simulink model "model"  (R2023a)
settings: Solver=VariableStepAuto  StartTime=0.0  StopTime=10  RelTol=1e-3
settings Model: Creator=grill  LastModifiedBy=grill

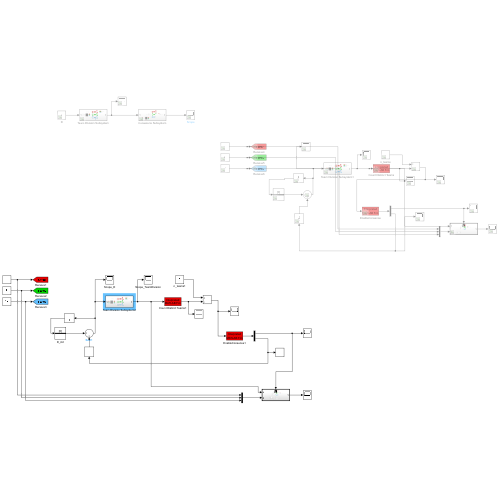
[thumbnail: Simulink's stored preview of the top-level diagram]
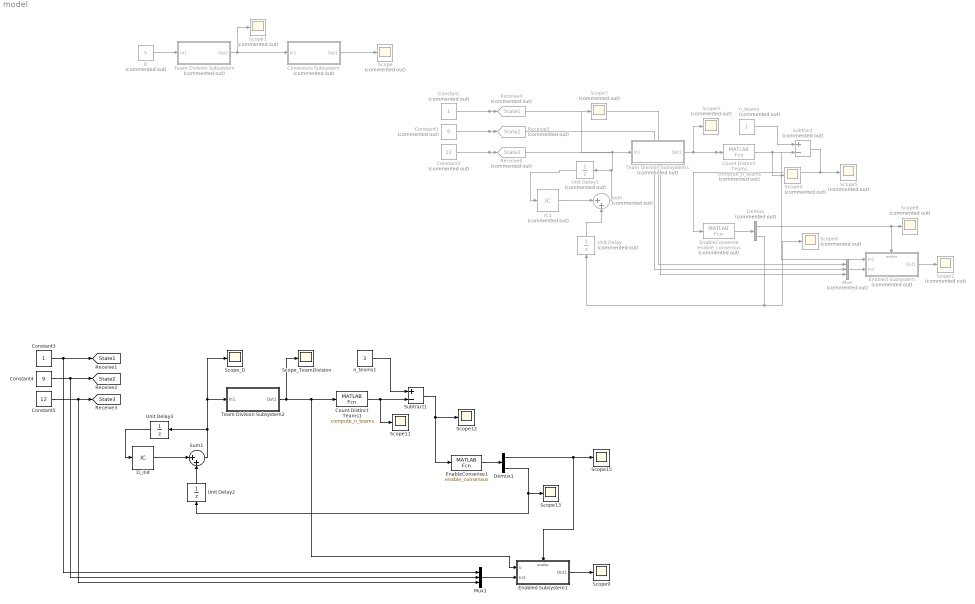
== system model ==
  " Receive4" : Goto  Commented=on  GotoTag=State1  TagVisibility=global
  " Receive5" : Goto  Commented=on  GotoTag=State2  TagVisibility=global
  " Receive6" : Goto  Commented=on  GotoTag=State3  TagVisibility=global
  Consesuns Subsystem : Subsystem  Commented=on
  Constant : Constant  Commented=on
  Constant1 : Constant  Commented=on  Value=9
  Constant2 : Constant  Commented=on  Value=12
  Constant3 : Constant
  Constant4 : Constant  Value=9
  Constant5 : Constant  Value=12
  Count Distinct Teams : MATLABFcn  Commented=on  MATLABFcn=compute_n_teams  OutputDimensions=1
  Count Distinct Teams1 : MATLABFcn  MATLABFcn=compute_n_teams  OutputDimensions=1
  D : Constant  Commented=on  Value=5
  D_init : InitialCondition  Value=0
  Demux : Demux  Commented=on  Outputs=2
  Demux1 : Demux  Outputs=2
  EnableConsense : MATLABFcn  Commented=on  MATLABFcn=enable_consensus  OutputDimensions=2
  EnableConsense1 : MATLABFcn  MATLABFcn=enable_consensus  OutputDimensions=2
  Enabled Subsystem : Subsystem  Commented=on  TreatAsAtomicUnit=on
  Enabled Subsystem1 : Subsystem  TreatAsAtomicUnit=on
  IC1 : InitialCondition  Commented=on  Value=0
  Mux : Mux  Commented=on  Inputs=3
  Mux1 : Mux  Inputs=3
  Scope{,1..8} (9 alike) : Scope  Commented=on
  Scope{9,11..13,15} (5 alike) : Scope
  Scope_D : Scope
  Scope_TeamDivision : Scope
  Subtract : Sum  Commented=on  Inputs=+-
  Subtract1 : Sum  Inputs=+-
  Sum : Sum  Commented=on  Inputs=|++
  Sum1 : Sum  Inputs=|++
  Team Division Subsystem : Subsystem  Commented=on
  Team Division Subsystem1 : Subsystem  Commented=on
  Team Division Subsystem2 : Subsystem
  Unit Delay : UnitDelay  Commented=on  SampleTime=-1  HasFrameUpgradeWarning=on
  Unit Delay1 : UnitDelay  Commented=on  SampleTime=-1  HasFrameUpgradeWarning=on
  Unit Delay2 : UnitDelay  SampleTime=-1  HasFrameUpgradeWarning=on
  Unit Delay3 : UnitDelay  SampleTime=-1  HasFrameUpgradeWarning=on
  n_teams : Constant  Commented=on
  n_teams1 : Constant  Value=3
  tag scope: State1=global, State2=global, State3=global
  wires:
  D/1 -> Team Division Subsystem/1(In1)
  Consesuns Subsystem/1(Out1) -> Scope/1
  Constant/1 -> Mux/1, " Receive4"/1
  Constant1/1 -> Mux/2, " Receive5"/1
  Constant2/1 -> Mux/3, " Receive6"/1
  Team Division Subsystem/1(Out1) -> Scope1/1, Consesuns Subsystem/1(In1)
  Mux/1 -> Enabled Subsystem/2(In2)
  n_teams/1 -> Subtract/1
  Subtract/1 -> Scope5/1, EnableConsense/1
  Count Distinct Teams/1 -> Scope4/1, Subtract/2
  Demux/2 -> Scope6/1, Unit Delay/1
  Team Division Subsystem1/1(Out1) -> Enabled Subsystem/1(In1), Count Distinct Teams/1, Scope3/1
  Unit Delay/1 -> Sum/2
  Sum/1 -> Team Division Subsystem1/1(In1), Scope7/1, Unit Delay1/1
  IC1/1 -> Sum/1
  Unit Delay1/1 -> IC1/1
  EnableConsense/1 -> Demux/1
  Demux/1 -> Scope8/1, Enabled Subsystem/Enable
  Enabled Subsystem/1(Out1) -> Scope2/1
  Demux1/1 -> Scope15/1, Enabled Subsystem1/Enable
  Enabled Subsystem1/1(Out1) -> Scope9/1
  D_init/1 -> Sum1/1
  Unit Delay3/1 -> D_init/1
  EnableConsense1/1 -> Demux1/1
  Team Division Subsystem2/1(Out1) -> Enabled Subsystem1/1(u), Count Distinct Teams1/1, Scope_TeamDivision/1
  Unit Delay2/1 -> Sum1/2
  Constant5/1 -> [State3], Mux1/3
  Constant4/1 -> Mux1/2, [State2]
  Sum1/1 -> Team Division Subsystem2/1(In1), Scope_D/1, Unit Delay3/1
  Subtract1/1 -> EnableConsense1/1, Scope12/1
  Constant3/1 -> [State1], Mux1/1
  n_teams1/1 -> Subtract1/1
  Mux1/1 -> Enabled Subsystem1/2(In2)
  Count Distinct Teams1/1 -> Scope11/1, Subtract1/2
  Demux1/2 -> Unit Delay2/1, Scope13/1

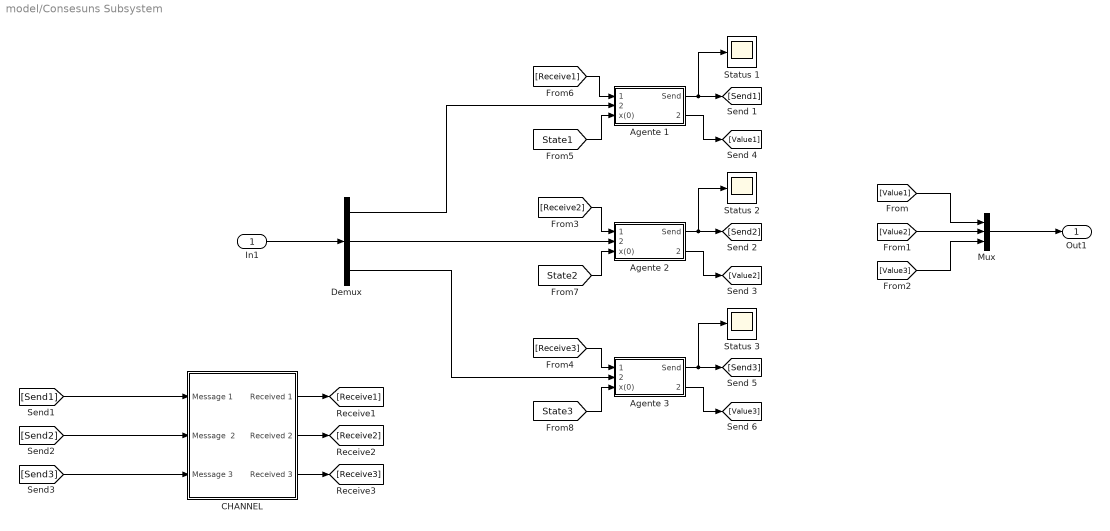
== system model/Consesuns Subsystem ==
  In1 : Inport
  Agente 1 : Subsystem
  Agente 2 : Subsystem
  Agente 3 : Subsystem
  CHANNEL : Subsystem
  Demux : Demux  Outputs=3
  Mux : Mux  Inputs=3
  Status 1 : Scope
  Status 2 : Scope
  Status 3 : Scope
  Out1 : Outport
  wires:
  Agente 1/1(Send) -> [Send1], Status 1/1
  In1/1 -> Demux/1
  Mux/1 -> Out1/1
  [Value3] -> Mux/3
  [Value2] -> Mux/2
  [Value1] -> Mux/1
  Demux/1 -> Agente 1/2(team_id)
  Agente 1/2(ValuePort) -> [Value1]
  Agente 2/1(Send) -> [Send2], Status 2/1
  Demux/2 -> Agente 2/2(team_id)
  Agente 2/2(ValuePort) -> [Value2]
  Agente 3/1(Send) -> [Send3], Status 3/1
  Demux/3 -> Agente 3/2(team_id)
  Agente 3/2(ValuePort) -> [Value3]
  [Receive1] -> Agente 1/1(Receive)
  [Receive2] -> Agente 2/1(Receive)
  [Receive3] -> Agente 3/1(Receive)
  CHANNEL/2(Received 2) -> [Receive2]
  CHANNEL/1(Received 1) -> [Receive1]
  CHANNEL/3(Received 3) -> [Receive3]
  [State1] -> Agente 1/3(x(0))
  [State2] -> Agente 2/3(x(0))
  [State3] -> Agente 3/3(x(0))
  [Send3] -> CHANNEL/3(Message 3)
  [Send2] -> CHANNEL/2(Message  2)
  [Send1] -> CHANNEL/1(Message 1)

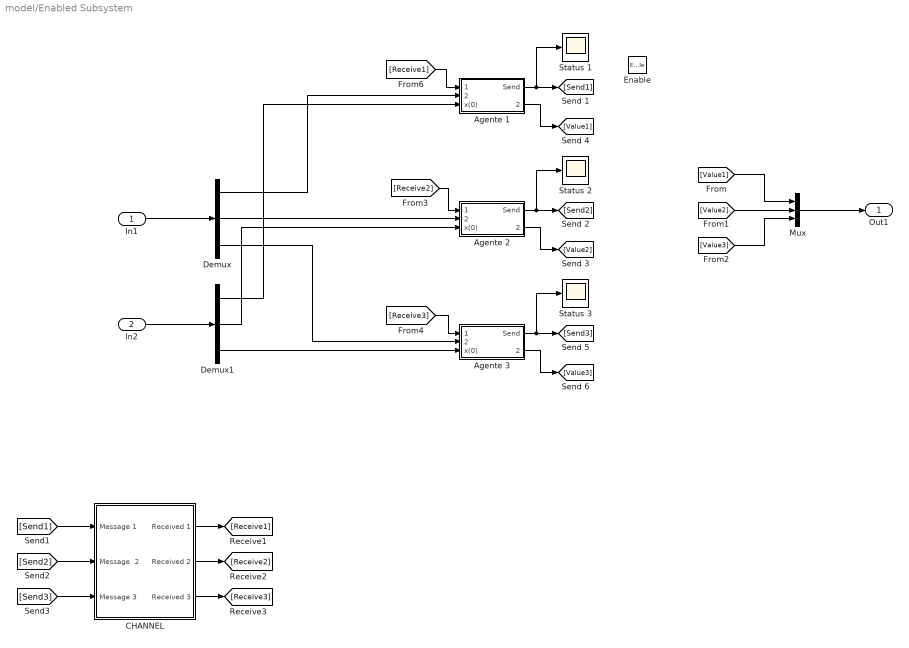
== system model/Enabled Subsystem ==
  In1 : Inport
  In2 : Inport  Port=2
  Enable : EnablePort
  Agente 1 : Subsystem
  Agente 2 : Subsystem
  Agente 3 : Subsystem
  CHANNEL : Subsystem
  Demux : Demux  Outputs=3
  Demux1 : Demux  Outputs=3
  Mux : Mux  Inputs=3
  Status 1 : Scope
  Status 2 : Scope
  Status 3 : Scope
  Out1 : Outport
  wires:
  Demux1/3 -> Agente 3/3(x(0))
  Demux1/1 -> Agente 1/3(x(0))
  Demux/2 -> Agente 2/2(team_id)
  Demux1/2 -> Agente 2/3(x(0))
  Agente 2/1(Send) -> [Send2], Status 2/1
  CHANNEL/3(Received 3) -> [Receive3]
  In1/1 -> Demux/1
  Agente 3/2(ValuePort) -> [Value3]
  [Value3] -> Mux/3
  Agente 2/2(ValuePort) -> [Value2]
  Agente 1/2(ValuePort) -> [Value1]
  [Receive2] -> Agente 2/1(Receive)
  [Receive3] -> Agente 3/1(Receive)
  CHANNEL/2(Received 2) -> [Receive2]
  In2/1 -> Demux1/1
  [Value1] -> Mux/1
  Mux/1 -> Out1/1
  [Send1] -> CHANNEL/1(Message 1)
  [Send2] -> CHANNEL/2(Message  2)
  [Send3] -> CHANNEL/3(Message 3)
  [Receive1] -> Agente 1/1(Receive)
  Demux/1 -> Agente 1/2(team_id)
  [Value2] -> Mux/2
  Agente 1/1(Send) -> [Send1], Status 1/1
  CHANNEL/1(Received 1) -> [Receive1]
  Demux/3 -> Agente 3/2(team_id)
  Agente 3/1(Send) -> [Send3], Status 3/1

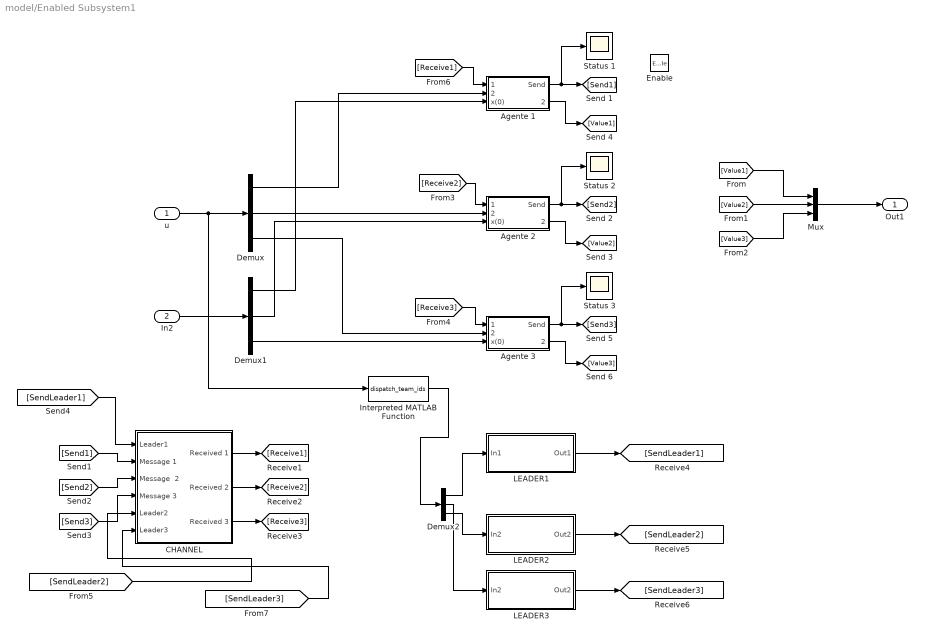
== system model/Enabled Subsystem1 ==
  u : Inport
  In2 : Inport  Port=2
  Enable : EnablePort
  Agente 1 : Subsystem
  Agente 2 : Subsystem
  Agente 3 : Subsystem
  CHANNEL : Subsystem
  Demux : Demux  Outputs=3
  Demux1 : Demux  Outputs=3
  Demux2 : Demux  Outputs=3
  Interpreted MATLAB Function : MATLABFcn  MATLABFcn=dispatch_team_ids  OutputDimensions=3
  LEADER1 : Subsystem
  LEADER2 : Subsystem
  LEADER3 : Subsystem
  Mux : Mux  Inputs=3
  Status 1 : Scope
  Status 2 : Scope
  Status 3 : Scope
  Out1 : Outport
  wires:
  Demux1/3 -> Agente 3/3(x(0))
  Demux1/1 -> Agente 1/3(x(0))
  Demux/2 -> Agente 2/2(team_id)
  Demux1/2 -> Agente 2/3(x(0))
  Agente 2/1(Send) -> [Send2], Status 2/1
  CHANNEL/3(Received 3) -> [Receive3]
  u/1 -> Interpreted MATLAB Function/1, Demux/1
  Agente 3/2(ValuePort) -> [Value3]
  [Value3] -> Mux/3
  Agente 2/2(ValuePort) -> [Value2]
  Agente 1/2(ValuePort) -> [Value1]
  [Receive2] -> Agente 2/1(Receive)
  [Receive3] -> Agente 3/1(Receive)
  CHANNEL/2(Received 2) -> [Receive2]
  In2/1 -> Demux1/1
  [Value1] -> Mux/1
  Mux/1 -> Out1/1
  [Send1] -> CHANNEL/2(Message 1)
  [Send2] -> CHANNEL/3(Message  2)
  [Send3] -> CHANNEL/4(Message 3)
  [Receive1] -> Agente 1/1(Receive)
  Demux/1 -> Agente 1/2(team_id)
  [Value2] -> Mux/2
  Agente 1/1(Send) -> [Send1], Status 1/1
  CHANNEL/1(Received 1) -> [Receive1]
  Demux/3 -> Agente 3/2(team_id)
  Agente 3/1(Send) -> [Send3], Status 3/1
  LEADER1/1(Out1) -> [SendLeader1]
  [SendLeader1] -> CHANNEL/1(Leader1)
  LEADER2/1(Out2) -> [SendLeader2]
  [SendLeader2] -> CHANNEL/5(Leader2)
  Interpreted MATLAB Function/1 -> Demux2/1
  Demux2/1 -> LEADER1/1(In1)
  Demux2/3 -> LEADER2/1(In2)
  LEADER3/1(Out2) -> [SendLeader3]
  Demux2/2 -> LEADER3/1(In2)
  [SendLeader3] -> CHANNEL/6(Leader3)

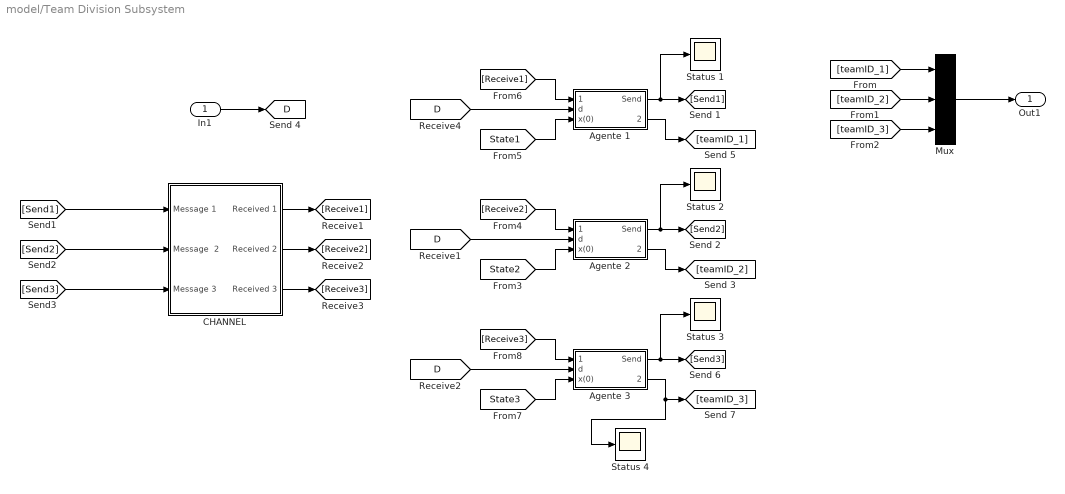
== system model/Team Division Subsystem ==
  In1 : Inport
  Agente 1 : Subsystem
  Agente 2 : Subsystem
  Agente 3 : Subsystem
  CHANNEL : Subsystem
  Mux : Mux  Inputs=3
  Status {1..4} (4 alike) : Scope
  Out1 : Outport
  tag scope: D=global
  wires:
  Agente 1/1(Send) -> [Send1], Status 1/1
  [D] -> Agente 1/2(d)
  Mux/1 -> Out1/1
  Agente 1/2(TeamPort) -> [teamID_1]
  [teamID_3] -> Mux/3
  [teamID_2] -> Mux/2
  [teamID_1] -> Mux/1
  In1/1 -> [D]
  [Receive1] -> Agente 1/1(Receive)
  [State1] -> Agente 1/3(x(0))
  Agente 2/2(TeamPort) -> [teamID_2]
  [State2] -> Agente 2/3(x(0))
  Agente 2/1(Send) -> [Send2], Status 2/1
  [D] -> Agente 2/2(d)
  [Receive2] -> Agente 2/1(Receive)
  Agente 3/2(TeamPort) -> Status 4/1, [teamID_3]
  [State3] -> Agente 3/3(x(0))
  Agente 3/1(Send) -> [Send3], Status 3/1
  [D] -> Agente 3/2(d)
  [Receive3] -> Agente 3/1(Receive)
  CHANNEL/2(Received 2) -> [Receive2]
  CHANNEL/1(Received 1) -> [Receive1]
  CHANNEL/3(Received 3) -> [Receive3]
  [Send1] -> CHANNEL/1(Message 1)
  [Send2] -> CHANNEL/2(Message  2)
  [Send3] -> CHANNEL/3(Message 3)

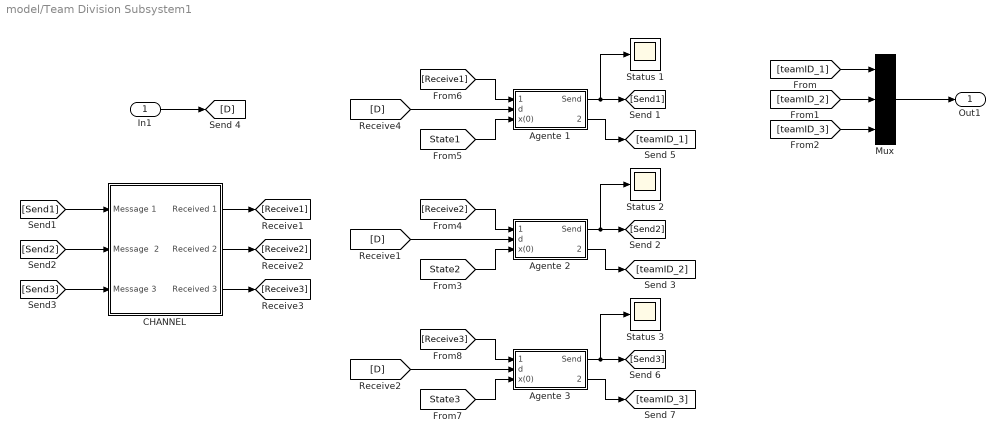
== system model/Team Division Subsystem1 ==
  In1 : Inport
  Agente 1 : Subsystem
  Agente 2 : Subsystem
  Agente 3 : Subsystem
  CHANNEL : Subsystem
  Mux : Mux  Inputs=3
  Status 1 : Scope
  Status 2 : Scope
  Status 3 : Scope
  Out1 : Outport
  wires:
  Agente 1/1(Send) -> [Send1], Status 1/1
  [D] -> Agente 1/2(d)
  Mux/1 -> Out1/1
  Agente 1/2(TeamPort) -> [teamID_1]
  [teamID_3] -> Mux/3
  [teamID_2] -> Mux/2
  [teamID_1] -> Mux/1
  In1/1 -> [D]
  [Receive1] -> Agente 1/1(Receive)
  [State1] -> Agente 1/3(x(0))
  Agente 2/2(TeamPort) -> [teamID_2]
  [State2] -> Agente 2/3(x(0))
  Agente 2/1(Send) -> [Send2], Status 2/1
  [D] -> Agente 2/2(d)
  [Receive2] -> Agente 2/1(Receive)
  Agente 3/2(TeamPort) -> [teamID_3]
  [State3] -> Agente 3/3(x(0))
  Agente 3/1(Send) -> [Send3], Status 3/1
  [D] -> Agente 3/2(d)
  [Receive3] -> Agente 3/1(Receive)
  CHANNEL/2(Received 2) -> [Receive2]
  [Send1] -> CHANNEL/1(Message 1)
  CHANNEL/1(Received 1) -> [Receive1]
  [Send2] -> CHANNEL/2(Message  2)
  [Send3] -> CHANNEL/3(Message 3)
  CHANNEL/3(Received 3) -> [Receive3]

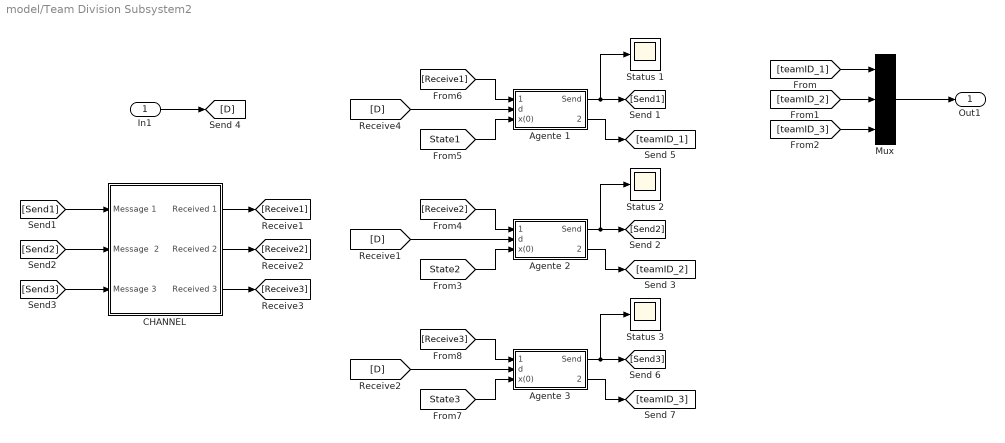
== system model/Team Division Subsystem2 ==
  In1 : Inport
  Agente 1 : Subsystem
  Agente 2 : Subsystem
  Agente 3 : Subsystem
  CHANNEL : Subsystem
  Mux : Mux  Inputs=3
  Status 1 : Scope
  Status 2 : Scope
  Status 3 : Scope
  Out1 : Outport
  wires:
  Agente 1/1(Send) -> [Send1], Status 1/1
  [D] -> Agente 1/2(d)
  Mux/1 -> Out1/1
  Agente 1/2(TeamPort) -> [teamID_1]
  [teamID_3] -> Mux/3
  [teamID_2] -> Mux/2
  [teamID_1] -> Mux/1
  In1/1 -> [D]
  [Receive1] -> Agente 1/1(Receive)
  [State1] -> Agente 1/3(x(0))
  Agente 2/2(TeamPort) -> [teamID_2]
  [State2] -> Agente 2/3(x(0))
  Agente 2/1(Send) -> [Send2], Status 2/1
  [D] -> Agente 2/2(d)
  [Receive2] -> Agente 2/1(Receive)
  Agente 3/2(TeamPort) -> [teamID_3]
  [State3] -> Agente 3/3(x(0))
  Agente 3/1(Send) -> [Send3], Status 3/1
  [D] -> Agente 3/2(d)
  [Receive3] -> Agente 3/1(Receive)
  CHANNEL/2(Received 2) -> [Receive2]
  [Send1] -> CHANNEL/1(Message 1)
  CHANNEL/1(Received 1) -> [Receive1]
  [Send2] -> CHANNEL/2(Message  2)
  [Send3] -> CHANNEL/3(Message 3)
  CHANNEL/3(Received 3) -> [Receive3]

== system model/Consesuns Subsystem/Agente 1 ==
  Receive : Inport
  team_id : Inport  Port=2
  x(0) : Inport  Port=3
  Agente 1 : MATLABFcn  MATLABFcn=consensus  OutputDimensions=2
  Demux : Demux  Outputs=2
  Integrator : Integrator  InitialConditionSource=external  InitialCondition=1
  Mux : Mux  Inputs=2
  Mux1 : Mux  Inputs=3
  Scope : Scope
  input_fnc Display : Display
  output_fnc Display : Display
  Send : Outport  VectorParamsAs1DForOutWhenUnconnected=off
  ValuePort : Outport  Port=2
  wires:
  Receive/1 -> Mux1/1, Scope/1
  team_id/1 -> Mux1/2
  Agente 1/1 -> output_fnc Display/1, Demux/1
  Mux/1 -> Send/1
  Demux/1 -> Mux/1
  Mux1/1 -> input_fnc Display/1, Agente 1/1
  Demux/2 -> Integrator/1
  Integrator/1 -> ValuePort/1, Mux1/3, Mux/2
  x(0)/1 -> Integrator/2

== system model/Consesuns Subsystem/Agente 2 ==
  Receive : Inport
  team_id : Inport  Port=2
  x(0) : Inport  Port=3
  Agente 1 : MATLABFcn  MATLABFcn=consensus  OutputDimensions=2
  Demux : Demux  Outputs=2
  Integrator : Integrator  InitialConditionSource=external  InitialCondition=1
  Mux : Mux  Inputs=2
  Mux1 : Mux  Inputs=3
  Scope : Scope
  input_fnc Display : Display
  output_fnc Display : Display
  Send : Outport  VectorParamsAs1DForOutWhenUnconnected=off
  ValuePort : Outport  Port=2
  wires:
  Receive/1 -> Mux1/1, Scope/1
  team_id/1 -> Mux1/2
  Agente 1/1 -> output_fnc Display/1, Demux/1
  Mux/1 -> Send/1
  Demux/1 -> Mux/1
  Mux1/1 -> input_fnc Display/1, Agente 1/1
  Demux/2 -> Integrator/1
  Integrator/1 -> ValuePort/1, Mux1/3, Mux/2
  x(0)/1 -> Integrator/2

== system model/Consesuns Subsystem/Agente 3 ==
  Receive : Inport
  team_id : Inport  Port=2
  x(0) : Inport  Port=3
  Agente 1 : MATLABFcn  MATLABFcn=consensus  OutputDimensions=2
  Demux : Demux  Outputs=2
  Integrator : Integrator  InitialConditionSource=external  InitialCondition=1
  Mux : Mux  Inputs=2
  Mux1 : Mux  Inputs=3
  Scope : Scope
  input_fnc Display : Display
  output_fnc Display : Display
  Send : Outport  VectorParamsAs1DForOutWhenUnconnected=off
  ValuePort : Outport  Port=2
  wires:
  Receive/1 -> Mux1/1, Scope/1
  team_id/1 -> Mux1/2
  Agente 1/1 -> output_fnc Display/1, Demux/1
  Mux/1 -> Send/1
  Demux/1 -> Mux/1
  Mux1/1 -> input_fnc Display/1, Agente 1/1
  Demux/2 -> Integrator/1
  Integrator/1 -> ValuePort/1, Mux1/3, Mux/2
  x(0)/1 -> Integrator/2

== system model/Consesuns Subsystem/CHANNEL ==
  Message 1 : Inport
  Message  2 : Inport  Port=2
  Message 3 : Inport  Port=3
  Mux : Mux  Inputs=2
  Mux1 : Mux  Inputs=2
  Mux2 : Mux  Inputs=2
  Received 1 : Outport  VectorParamsAs1DForOutWhenUnconnected=off
  Received 2 : Outport  Port=2  VectorParamsAs1DForOutWhenUnconnected=off
  Received 3 : Outport  Port=3  VectorParamsAs1DForOutWhenUnconnected=off
  wires:
  Mux2/1 -> Received 3/1
  Mux1/1 -> Received 2/1
  Mux/1 -> Received 1/1
  Message 1/1 -> Mux2/1, Mux1/1
  Message  2/1 -> Mux2/2, Mux/1
  Message 3/1 -> Mux/2, Mux1/2

== system model/Enabled Subsystem/Agente 1 ==
  Receive : Inport
  team_id : Inport  Port=2
  x(0) : Inport  Port=3
  Agente 1 : MATLABFcn  MATLABFcn=consensus  OutputDimensions=2
  Demux : Demux  Outputs=2
  Integrator : Integrator  InitialConditionSource=external  InitialCondition=1
  Mux : Mux  Inputs=2
  Mux1 : Mux  Inputs=3
  Scope : Scope
  input_fnc Display : Display
  output_fnc Display : Display
  Send : Outport  VectorParamsAs1DForOutWhenUnconnected=off
  ValuePort : Outport  Port=2
  wires:
  Receive/1 -> Mux1/1, Scope/1
  team_id/1 -> Mux1/2
  Agente 1/1 -> output_fnc Display/1, Demux/1
  Mux/1 -> Send/1
  Demux/1 -> Mux/1
  Mux1/1 -> input_fnc Display/1, Agente 1/1
  Demux/2 -> Integrator/1
  Integrator/1 -> ValuePort/1, Mux1/3, Mux/2
  x(0)/1 -> Integrator/2

== system model/Enabled Subsystem/Agente 2 ==
  Receive : Inport
  team_id : Inport  Port=2
  x(0) : Inport  Port=3
  Agente 1 : MATLABFcn  MATLABFcn=consensus  OutputDimensions=2
  Demux : Demux  Outputs=2
  Integrator : Integrator  InitialConditionSource=external  InitialCondition=1
  Mux : Mux  Inputs=2
  Mux1 : Mux  Inputs=3
  Scope : Scope
  input_fnc Display : Display
  output_fnc Display : Display
  Send : Outport  VectorParamsAs1DForOutWhenUnconnected=off
  ValuePort : Outport  Port=2
  wires:
  Receive/1 -> Mux1/1, Scope/1
  team_id/1 -> Mux1/2
  Agente 1/1 -> output_fnc Display/1, Demux/1
  Mux/1 -> Send/1
  Demux/1 -> Mux/1
  Mux1/1 -> input_fnc Display/1, Agente 1/1
  Demux/2 -> Integrator/1
  Integrator/1 -> ValuePort/1, Mux1/3, Mux/2
  x(0)/1 -> Integrator/2

== system model/Enabled Subsystem/Agente 3 ==
  Receive : Inport
  team_id : Inport  Port=2
  x(0) : Inport  Port=3
  Agente 1 : MATLABFcn  MATLABFcn=consensus  OutputDimensions=2
  Demux : Demux  Outputs=2
  Integrator : Integrator  InitialConditionSource=external  InitialCondition=1
  Mux : Mux  Inputs=2
  Mux1 : Mux  Inputs=3
  Scope : Scope
  input_fnc Display : Display
  output_fnc Display : Display
  Send : Outport  VectorParamsAs1DForOutWhenUnconnected=off
  ValuePort : Outport  Port=2
  wires:
  Receive/1 -> Mux1/1, Scope/1
  team_id/1 -> Mux1/2
  Agente 1/1 -> output_fnc Display/1, Demux/1
  Mux/1 -> Send/1
  Demux/1 -> Mux/1
  Mux1/1 -> input_fnc Display/1, Agente 1/1
  Demux/2 -> Integrator/1
  Integrator/1 -> ValuePort/1, Mux1/3, Mux/2
  x(0)/1 -> Integrator/2

== system model/Enabled Subsystem/CHANNEL ==
  Message 1 : Inport
  Message  2 : Inport  Port=2
  Message 3 : Inport  Port=3
  Mux : Mux  Inputs=2
  Mux1 : Mux  Inputs=2
  Mux2 : Mux  Inputs=2
  Received 1 : Outport  VectorParamsAs1DForOutWhenUnconnected=off
  Received 2 : Outport  Port=2  VectorParamsAs1DForOutWhenUnconnected=off
  Received 3 : Outport  Port=3  VectorParamsAs1DForOutWhenUnconnected=off
  wires:
  Mux2/1 -> Received 3/1
  Mux1/1 -> Received 2/1
  Mux/1 -> Received 1/1
  Message 1/1 -> Mux2/1, Mux1/1
  Message  2/1 -> Mux2/2, Mux/1
  Message 3/1 -> Mux/2, Mux1/2

== system model/Enabled Subsystem1/Agente 1 ==
  Receive : Inport
  team_id : Inport  Port=2
  x(0) : Inport  Port=3
  Agente 1 : MATLABFcn  MATLABFcn=consensus  OutputDimensions=2
  Demux : Demux  Outputs=2
  Integrator : Integrator  InitialConditionSource=external  InitialCondition=1
  Mux : Mux  Inputs=2
  Mux1 : Mux  Inputs=3
  Scope : Scope
  input_fnc Display : Display
  output_fnc Display : Display
  Send : Outport  VectorParamsAs1DForOutWhenUnconnected=off
  ValuePort : Outport  Port=2
  wires:
  Receive/1 -> Mux1/1, Scope/1
  team_id/1 -> Mux1/2
  Agente 1/1 -> output_fnc Display/1, Demux/1
  Mux/1 -> Send/1
  Demux/1 -> Mux/1
  Mux1/1 -> input_fnc Display/1, Agente 1/1
  Demux/2 -> Integrator/1
  Integrator/1 -> ValuePort/1, Mux1/3, Mux/2
  x(0)/1 -> Integrator/2

== system model/Enabled Subsystem1/Agente 2 ==
  Receive : Inport
  team_id : Inport  Port=2
  x(0) : Inport  Port=3
  Agente 1 : MATLABFcn  MATLABFcn=consensus  OutputDimensions=2
  Demux : Demux  Outputs=2
  Integrator : Integrator  InitialConditionSource=external  InitialCondition=1
  Mux : Mux  Inputs=2
  Mux1 : Mux  Inputs=3
  Scope : Scope
  input_fnc Display : Display
  output_fnc Display : Display
  Send : Outport  VectorParamsAs1DForOutWhenUnconnected=off
  ValuePort : Outport  Port=2
  wires:
  Receive/1 -> Mux1/1, Scope/1
  team_id/1 -> Mux1/2
  Agente 1/1 -> output_fnc Display/1, Demux/1
  Mux/1 -> Send/1
  Demux/1 -> Mux/1
  Mux1/1 -> input_fnc Display/1, Agente 1/1
  Demux/2 -> Integrator/1
  Integrator/1 -> ValuePort/1, Mux1/3, Mux/2
  x(0)/1 -> Integrator/2

== system model/Enabled Subsystem1/Agente 3 ==
  Receive : Inport
  team_id : Inport  Port=2
  x(0) : Inport  Port=3
  Agente 1 : MATLABFcn  MATLABFcn=consensus  OutputDimensions=2
  Demux : Demux  Outputs=2
  Integrator : Integrator  InitialConditionSource=external  InitialCondition=1
  Mux : Mux  Inputs=2
  Mux1 : Mux  Inputs=3
  Scope : Scope
  input_fnc Display : Display
  output_fnc Display : Display
  Send : Outport  VectorParamsAs1DForOutWhenUnconnected=off
  ValuePort : Outport  Port=2
  wires:
  Receive/1 -> Mux1/1, Scope/1
  team_id/1 -> Mux1/2
  Agente 1/1 -> output_fnc Display/1, Demux/1
  Mux/1 -> Send/1
  Demux/1 -> Mux/1
  Mux1/1 -> input_fnc Display/1, Agente 1/1
  Demux/2 -> Integrator/1
  Integrator/1 -> ValuePort/1, Mux1/3, Mux/2
  x(0)/1 -> Integrator/2

== system model/Enabled Subsystem1/CHANNEL ==
  Leader1 : Inport
  Message 1 : Inport  Port=2
  Message  2 : Inport  Port=3
  Message 3 : Inport  Port=4
  Leader2 : Inport  Port=5
  Leader3 : Inport  Port=6
  Mux : Mux  Inputs=5
  Mux1 : Mux  Inputs=5
  Mux2 : Mux  Inputs=5
  Received 1 : Outport  VectorParamsAs1DForOutWhenUnconnected=off
  Received 2 : Outport  Port=2  VectorParamsAs1DForOutWhenUnconnected=off
  Received 3 : Outport  Port=3  VectorParamsAs1DForOutWhenUnconnected=off
  wires:
  Mux2/1 -> Received 3/1
  Mux1/1 -> Received 2/1
  Mux/1 -> Received 1/1
  Message 1/1 -> Mux2/4, Mux1/4
  Message  2/1 -> Mux2/5, Mux/4
  Message 3/1 -> Mux/5, Mux1/5
  Leader1/1 -> Mux2/1, Mux/1, Mux1/1
  Leader2/1 -> Mux2/2, Mux1/2, Mux/2
  Leader3/1 -> Mux2/3, Mux1/3, Mux/3

== system model/Enabled Subsystem1/LEADER1 ==
  In1 : Inport
  Constant : Constant  Value=20
  Mux : Mux  Inputs=2
  Out1 : Outport
  wires:
  In1/1 -> Mux/1
  Constant/1 -> Mux/2
  Mux/1 -> Out1/1

== system model/Enabled Subsystem1/LEADER2 ==
  In2 : Inport
  Constant : Constant  Value=40
  Mux : Mux  Inputs=2
  Out2 : Outport
  wires:
  In2/1 -> Mux/1
  Mux/1 -> Out2/1
  Constant/1 -> Mux/2

== system model/Enabled Subsystem1/LEADER3 ==
  In2 : Inport
  Constant : Constant  Value=60
  Mux : Mux  Inputs=2
  Out2 : Outport
  wires:
  In2/1 -> Mux/1
  Mux/1 -> Out2/1
  Constant/1 -> Mux/2

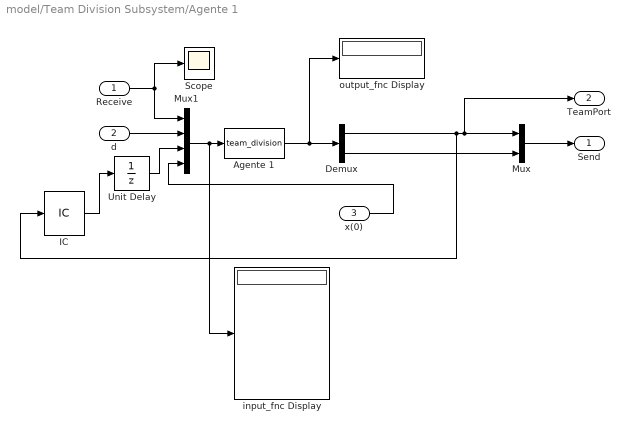
== system model/Team Division Subsystem/Agente 1 ==
  Receive : Inport
  d : Inport  Port=2
  x(0) : Inport  Port=3
  Agente 1 : MATLABFcn  MATLABFcn=team_division  OutputDimensions=2
  Demux : Demux  Outputs=2
  IC : InitialCondition  Value=1000
  Mux : Mux  Inputs=2
  Mux1 : Mux
  Scope : Scope
  Unit Delay : UnitDelay  SampleTime=-1  HasFrameUpgradeWarning=on
  input_fnc Display : Display
  output_fnc Display : Display
  Send : Outport  VectorParamsAs1DForOutWhenUnconnected=off
  TeamPort : Outport  Port=2
  wires:
  Receive/1 -> Mux1/1, Scope/1
  d/1 -> Mux1/2
  IC/1 -> Unit Delay/1
  Agente 1/1 -> output_fnc Display/1, Demux/1
  Mux/1 -> Send/1
  Mux1/1 -> input_fnc Display/1, Agente 1/1
  Demux/2 -> Mux/2
  x(0)/1 -> Mux1/4
  Demux/1 -> IC/1, TeamPort/1, Mux/1
  Unit Delay/1 -> Mux1/3

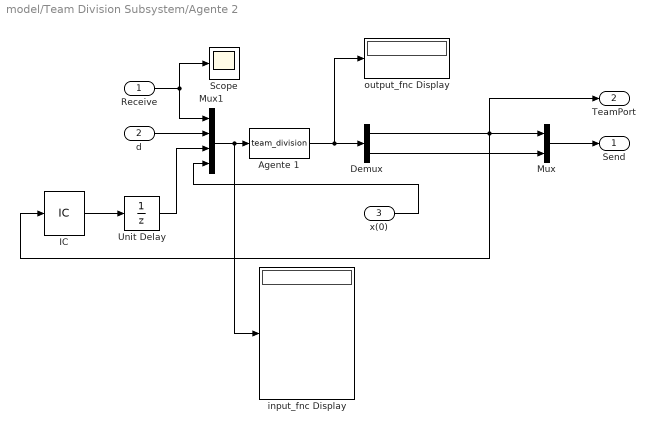
== system model/Team Division Subsystem/Agente 2 ==
  Receive : Inport
  d : Inport  Port=2
  x(0) : Inport  Port=3
  Agente 1 : MATLABFcn  MATLABFcn=team_division  OutputDimensions=2
  Demux : Demux  Outputs=2
  IC : InitialCondition  Value=1001
  Mux : Mux  Inputs=2
  Mux1 : Mux
  Scope : Scope
  Unit Delay : UnitDelay  SampleTime=-1  HasFrameUpgradeWarning=on
  input_fnc Display : Display
  output_fnc Display : Display
  Send : Outport  VectorParamsAs1DForOutWhenUnconnected=off
  TeamPort : Outport  Port=2
  wires:
  Receive/1 -> Mux1/1, Scope/1
  d/1 -> Mux1/2
  IC/1 -> Unit Delay/1
  Agente 1/1 -> output_fnc Display/1, Demux/1
  Mux/1 -> Send/1
  Mux1/1 -> input_fnc Display/1, Agente 1/1
  Demux/2 -> Mux/2
  x(0)/1 -> Mux1/4
  Demux/1 -> IC/1, TeamPort/1, Mux/1
  Unit Delay/1 -> Mux1/3

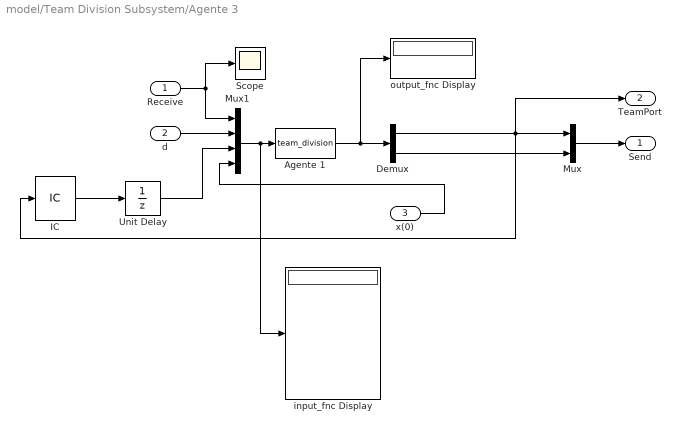
== system model/Team Division Subsystem/Agente 3 ==
  Receive : Inport
  d : Inport  Port=2
  x(0) : Inport  Port=3
  Agente 1 : MATLABFcn  MATLABFcn=team_division  OutputDimensions=2
  Demux : Demux  Outputs=2
  IC : InitialCondition  Value=1002
  Mux : Mux  Inputs=2
  Mux1 : Mux
  Scope : Scope
  Unit Delay : UnitDelay  SampleTime=-1  HasFrameUpgradeWarning=on
  input_fnc Display : Display
  output_fnc Display : Display
  Send : Outport  VectorParamsAs1DForOutWhenUnconnected=off
  TeamPort : Outport  Port=2
  wires:
  Receive/1 -> Mux1/1, Scope/1
  d/1 -> Mux1/2
  IC/1 -> Unit Delay/1
  Agente 1/1 -> output_fnc Display/1, Demux/1
  Mux/1 -> Send/1
  Mux1/1 -> input_fnc Display/1, Agente 1/1
  Demux/2 -> Mux/2
  x(0)/1 -> Mux1/4
  Demux/1 -> IC/1, TeamPort/1, Mux/1
  Unit Delay/1 -> Mux1/3

== system model/Team Division Subsystem/CHANNEL ==
  Message 1 : Inport
  Message  2 : Inport  Port=2
  Message 3 : Inport  Port=3
  Mux : Mux  Inputs=2
  Mux1 : Mux  Inputs=2
  Mux2 : Mux  Inputs=2
  Received 1 : Outport  VectorParamsAs1DForOutWhenUnconnected=off
  Received 2 : Outport  Port=2  VectorParamsAs1DForOutWhenUnconnected=off
  Received 3 : Outport  Port=3  VectorParamsAs1DForOutWhenUnconnected=off
  wires:
  Mux2/1 -> Received 3/1
  Mux1/1 -> Received 2/1
  Mux/1 -> Received 1/1
  Message 1/1 -> Mux2/1, Mux1/1
  Message  2/1 -> Mux2/2, Mux/1
  Message 3/1 -> Mux/2, Mux1/2

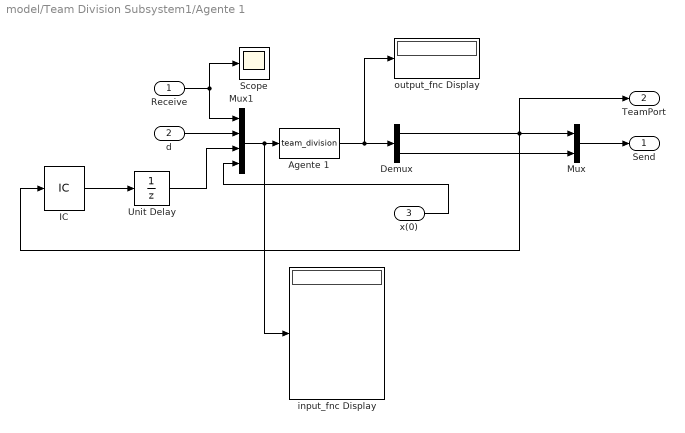
== system model/Team Division Subsystem1/Agente 1 ==
  Receive : Inport
  d : Inport  Port=2
  x(0) : Inport  Port=3
  Agente 1 : MATLABFcn  MATLABFcn=team_division  OutputDimensions=2
  Demux : Demux  Outputs=2
  IC : InitialCondition  Value=100
  Mux : Mux  Inputs=2
  Mux1 : Mux
  Scope : Scope
  Unit Delay : UnitDelay  SampleTime=-1  HasFrameUpgradeWarning=on
  input_fnc Display : Display
  output_fnc Display : Display
  Send : Outport  VectorParamsAs1DForOutWhenUnconnected=off
  TeamPort : Outport  Port=2
  wires:
  Receive/1 -> Mux1/1, Scope/1
  d/1 -> Mux1/2
  IC/1 -> Unit Delay/1
  Agente 1/1 -> output_fnc Display/1, Demux/1
  Mux/1 -> Send/1
  Mux1/1 -> input_fnc Display/1, Agente 1/1
  Demux/2 -> Mux/2
  x(0)/1 -> Mux1/4
  Demux/1 -> IC/1, TeamPort/1, Mux/1
  Unit Delay/1 -> Mux1/3

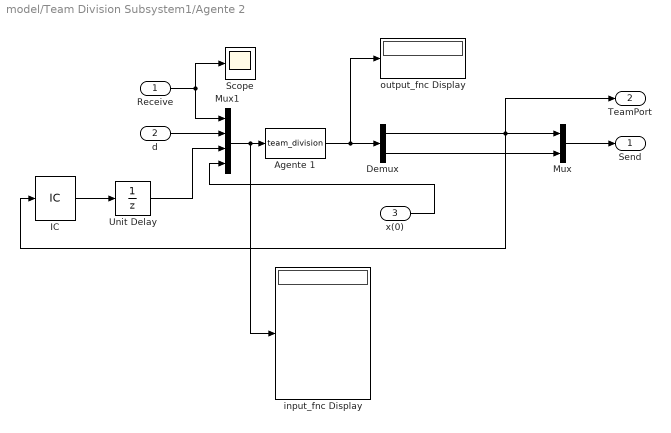
== system model/Team Division Subsystem1/Agente 2 ==
  Receive : Inport
  d : Inport  Port=2
  x(0) : Inport  Port=3
  Agente 1 : MATLABFcn  MATLABFcn=team_division  OutputDimensions=2
  Demux : Demux  Outputs=2
  IC : InitialCondition  Value=200
  Mux : Mux  Inputs=2
  Mux1 : Mux
  Scope : Scope
  Unit Delay : UnitDelay  SampleTime=-1  HasFrameUpgradeWarning=on
  input_fnc Display : Display
  output_fnc Display : Display
  Send : Outport  VectorParamsAs1DForOutWhenUnconnected=off
  TeamPort : Outport  Port=2
  wires:
  Receive/1 -> Mux1/1, Scope/1
  d/1 -> Mux1/2
  IC/1 -> Unit Delay/1
  Agente 1/1 -> output_fnc Display/1, Demux/1
  Mux/1 -> Send/1
  Mux1/1 -> input_fnc Display/1, Agente 1/1
  Demux/2 -> Mux/2
  x(0)/1 -> Mux1/4
  Demux/1 -> IC/1, TeamPort/1, Mux/1
  Unit Delay/1 -> Mux1/3

== system model/Team Division Subsystem1/Agente 3 ==
  Receive : Inport
  d : Inport  Port=2
  x(0) : Inport  Port=3
  Agente 1 : MATLABFcn  MATLABFcn=team_division  OutputDimensions=2
  Demux : Demux  Outputs=2
  IC : InitialCondition  Value=300
  Mux : Mux  Inputs=2
  Mux1 : Mux
  Scope : Scope
  Unit Delay : UnitDelay  SampleTime=-1  HasFrameUpgradeWarning=on
  input_fnc Display : Display
  output_fnc Display : Display
  Send : Outport  VectorParamsAs1DForOutWhenUnconnected=off
  TeamPort : Outport  Port=2
  wires:
  Receive/1 -> Mux1/1, Scope/1
  d/1 -> Mux1/2
  IC/1 -> Unit Delay/1
  Agente 1/1 -> output_fnc Display/1, Demux/1
  Mux/1 -> Send/1
  Mux1/1 -> input_fnc Display/1, Agente 1/1
  Demux/2 -> Mux/2
  x(0)/1 -> Mux1/4
  Demux/1 -> IC/1, TeamPort/1, Mux/1
  Unit Delay/1 -> Mux1/3

== system model/Team Division Subsystem1/CHANNEL ==
  Message 1 : Inport
  Message  2 : Inport  Port=2
  Message 3 : Inport  Port=3
  Mux : Mux  Inputs=2
  Mux1 : Mux  Inputs=2
  Mux2 : Mux  Inputs=2
  Received 1 : Outport  VectorParamsAs1DForOutWhenUnconnected=off
  Received 2 : Outport  Port=2  VectorParamsAs1DForOutWhenUnconnected=off
  Received 3 : Outport  Port=3  VectorParamsAs1DForOutWhenUnconnected=off
  wires:
  Mux2/1 -> Received 3/1
  Mux1/1 -> Received 2/1
  Mux/1 -> Received 1/1
  Message 1/1 -> Mux2/1, Mux1/1
  Message  2/1 -> Mux2/2, Mux/1
  Message 3/1 -> Mux/2, Mux1/2

== system model/Team Division Subsystem2/Agente 1 ==
  Receive : Inport
  d : Inport  Port=2
  x(0) : Inport  Port=3
  Agente 1 : MATLABFcn  MATLABFcn=team_division  OutputDimensions=2
  Demux : Demux  Outputs=2
  IC : InitialCondition  Value=100
  Mux : Mux  Inputs=2
  Mux1 : Mux
  Scope : Scope
  Unit Delay : UnitDelay  SampleTime=-1  HasFrameUpgradeWarning=on
  input_fnc Display : Display
  output_fnc Display : Display
  Send : Outport  VectorParamsAs1DForOutWhenUnconnected=off
  TeamPort : Outport  Port=2
  wires:
  Receive/1 -> Mux1/1, Scope/1
  d/1 -> Mux1/2
  IC/1 -> Unit Delay/1
  Agente 1/1 -> output_fnc Display/1, Demux/1
  Mux/1 -> Send/1
  Mux1/1 -> input_fnc Display/1, Agente 1/1
  Demux/2 -> Mux/2
  x(0)/1 -> Mux1/4
  Demux/1 -> IC/1, TeamPort/1, Mux/1
  Unit Delay/1 -> Mux1/3

== system model/Team Division Subsystem2/Agente 2 ==
  Receive : Inport
  d : Inport  Port=2
  x(0) : Inport  Port=3
  Agente 1 : MATLABFcn  MATLABFcn=team_division  OutputDimensions=2
  Demux : Demux  Outputs=2
  IC : InitialCondition  Value=200
  Mux : Mux  Inputs=2
  Mux1 : Mux
  Scope : Scope
  Unit Delay : UnitDelay  SampleTime=-1  HasFrameUpgradeWarning=on
  input_fnc Display : Display
  output_fnc Display : Display
  Send : Outport  VectorParamsAs1DForOutWhenUnconnected=off
  TeamPort : Outport  Port=2
  wires:
  Receive/1 -> Mux1/1, Scope/1
  d/1 -> Mux1/2
  IC/1 -> Unit Delay/1
  Agente 1/1 -> output_fnc Display/1, Demux/1
  Mux/1 -> Send/1
  Mux1/1 -> input_fnc Display/1, Agente 1/1
  Demux/2 -> Mux/2
  x(0)/1 -> Mux1/4
  Demux/1 -> IC/1, TeamPort/1, Mux/1
  Unit Delay/1 -> Mux1/3

== system model/Team Division Subsystem2/Agente 3 ==
  Receive : Inport
  d : Inport  Port=2
  x(0) : Inport  Port=3
  Agente 1 : MATLABFcn  MATLABFcn=team_division  OutputDimensions=2
  Demux : Demux  Outputs=2
  IC : InitialCondition  Value=300
  Mux : Mux  Inputs=2
  Mux1 : Mux
  Scope : Scope
  Unit Delay : UnitDelay  SampleTime=-1  HasFrameUpgradeWarning=on
  input_fnc Display : Display
  output_fnc Display : Display
  Send : Outport  VectorParamsAs1DForOutWhenUnconnected=off
  TeamPort : Outport  Port=2
  wires:
  Receive/1 -> Mux1/1, Scope/1
  d/1 -> Mux1/2
  IC/1 -> Unit Delay/1
  Agente 1/1 -> output_fnc Display/1, Demux/1
  Mux/1 -> Send/1
  Mux1/1 -> input_fnc Display/1, Agente 1/1
  Demux/2 -> Mux/2
  x(0)/1 -> Mux1/4
  Demux/1 -> IC/1, TeamPort/1, Mux/1
  Unit Delay/1 -> Mux1/3

== system model/Team Division Subsystem2/CHANNEL ==
  Message 1 : Inport
  Message  2 : Inport  Port=2
  Message 3 : Inport  Port=3
  Mux : Mux  Inputs=2
  Mux1 : Mux  Inputs=2
  Mux2 : Mux  Inputs=2
  Received 1 : Outport  VectorParamsAs1DForOutWhenUnconnected=off
  Received 2 : Outport  Port=2  VectorParamsAs1DForOutWhenUnconnected=off
  Received 3 : Outport  Port=3  VectorParamsAs1DForOutWhenUnconnected=off
  wires:
  Mux2/1 -> Received 3/1
  Mux1/1 -> Received 2/1
  Mux/1 -> Received 1/1
  Message 1/1 -> Mux2/1, Mux1/1
  Message  2/1 -> Mux2/2, Mux/1
  Message 3/1 -> Mux/2, Mux1/2
